simulink model "Forward_and_inverse_Both"  (R2024b)
settings: Solver=VariableStepAuto  StartTime=0.0  StopTime=7  MaxStep=0.005  RelTol=1e-3
model workspace: external: MATLAB File D:\OneDrive - itc.edu.kh\V4_robot_arm\Import_arm6\Test_Assembly_DataFile.m (data not in the file)
values from neighbouring files (symbols this model uses):
  Reach_max = max(REACH_MAX)    [Workspace_sample.m]
  Reach_min = max(REACH_MIN)    [Workspace_sample.m]
undefined symbols (not defined in the file or in its folder): DiscIntNeverNeededParam, initialPose, maxAngularAcc, maxAngularVel, maxLinearAcc, maxLinearVel, poseTol, smiData, Ts, wps1, X, Y, Z
libraries: sm_lib x140, nesl_utility x52, stmnucleolib x12, simulink x4, vrlib x2, vexcommonlib x2, robotcorelib x2
(part 6 of 6)

== matlab function Forward_and_inverse_Both/MATLAB Function ==
  data: Reach_min input; Reach_max input; x input; x_error input; x_out output; y input; y_error input; z input; z_error input; y_out output; z_out output; Out output
function [x_out, y_out, z_out, Out] = fcn(Reach_min, Reach_max, x, x_error, y, y_error, z, z_error)
    % Calculate the radial distance from origin
    Out = sqrt(x^2 + y^2 + z^2);

    % Check conditions for updating outputs
    if Out > Reach_min || Out < Reach_max || x == 0 && y == 0
        % Update outputs only if Out is within bounds and x, y = 0
        x_out = x;
        y_out = y;
        z_out = z;
    else
        % Retain previous outputs or use error positions
        x_out = x_error;
        y_out = y_error;
        z_out = z_error;
    end
end

== matlab function Forward_and_inverse_Both/Flip the state of a button1/MATLAB Function1 ==
  data: y output; X input; delta input; n input; error output
function [y , error] = fcn(X,delta,n)

    if X == 1 && n <= 2
        delta = 0;
        n = n + 1;
    elseif X == 1 && n > 2
        delta = 0;
        n = 0;
    elseif X == 0
        n = 0;
        delta = 1;
    end
    y = delta;
    error = n;
end

== matlab function Forward_and_inverse_Both/Set Delta for the joint movement more Delta, faster the movement1/ speed setting ==
  data: O input; Tri input; y output; delta input
function y = fcn(O,Tri,delta)

    if O == 1 && Tri ==0 && delta <= 0.1
        delta = delta + 0.025;
    elseif Tri == 1 && O == 0 && delta >= 0.025
        delta = delta - 0.025;
    else
    end
    y = delta;
end

== matlab function Forward_and_inverse_Both/Set Joint position to where it were left off1/Joint3 ==
  data: pos input; posfinal output; pos_prev input; delta input
function posfinal = fcn(pos,pos_prev,delta)

if pos > 0        %%In case of clockwise rotation
    posc = pos_prev + abs(delta);
elseif pos < 0    %%In case of counter clockwise rotation
    posc = pos_prev - abs(delta);
else               %%Stay still if there's no input
    posc = pos_prev;
end

if posc <= 1 && posc >= -1.2 %%The joint only update its position if it stays within this range
    posfinal = posc;
else
    posfinal = pos_prev;
end

== matlab function Forward_and_inverse_Both/Set Joint position to where it were left off1/Joint4 ==
  data: pos input; posfinal output; pos_prev input; delta input
function posfinal = fcn(pos,pos_prev,delta)

if pos > 0        %%In case of clockwise rotation
    posc = pos_prev + abs(delta);
elseif pos < 0    %%In case of counter clockwise rotation
    posc = pos_prev - abs(delta);
else               %%Stay still if there's no input
    posc = pos_prev;
end

if posc <= 1 && posc >= -1.2 %%The joint only update its position if it stays within this range
    posfinal = posc;
else
    posfinal = pos_prev;
end

== matlab function Forward_and_inverse_Both/Set Joint position to where it were left off1/MATLAB Function2 ==
  data: delta input; n input; y output; pos input; pos_prev input
function y = fcn(delta,n,pos,pos_prev)
if n == 0 && pos > 0
    pos = max(0,pos_prev - abs(delta));
elseif n == 0 && pos < 0
    pos = min(0,pos_prev + abs(delta));
end
y = pos;

== matlab function Forward_and_inverse_Both/Set Joint position to where it were left off1/MATLAB Function3 ==
  data: delta input; n input; y output; pos input; pos_prev input
function y = fcn(delta,n,pos,pos_prev)
if n == 0 && pos > 0
    pos = max(0,pos_prev - abs(delta));
elseif n == 0 && pos < 0
    pos = min(0,pos_prev + abs(delta));
end
y = pos;

== matlab function Forward_and_inverse_Both/Set Joint position to where it were left off1/limit J2 & J3 so that it won't collide with itself/Joint1 ==
  data: pos input; posfinal output; pos_prev input; delta input
function posfinal = fcn(pos,pos_prev,delta)

if pos > 0        %%In case of clockwise rotation
    posc = pos_prev + abs(delta);
elseif pos < 0    %%In case of counter clockwise rotation
    posc = pos_prev - abs(delta);
else               %%Stay still if there's no input
    posc = pos_prev;
end

if posc <= 1 && posc >= -1.2 %%The joint only update its position if it stays within this range
    posfinal = posc;
else
    posfinal = pos_prev;
end

== matlab function Forward_and_inverse_Both/Set Joint position to where it were left off1/limit J2 & J3 so that it won't collide with itself/Joint2 ==
  data: pos input; delta input; posfinal output; pos_prev input
function posfinal = fcn(pos,delta,pos_prev)

if pos > 0        %%In case of clockwise rotation
    posc = pos_prev + abs(delta);
elseif pos < 0    %%In case of counter clockwise rotation
    posc = pos_prev - abs(delta);
else               %%Stay still if there's no input
    posc = pos_prev;
end

if posc <= 1 && posc >= -1.2 %%The joint only update its position if it stays within this range
    posfinal = posc;
else
    posfinal = pos_prev;
end

== matlab function Forward_and_inverse_Both/Set Joint position to where it were left off1/limit J2 & J3 so that it won't collide with itself/MATLAB Function ==
  data: delta input; n input; y output; pos input; pos_prev input
function y = fcn(delta,n,pos,pos_prev)
if n == 0 && pos > 0
    pos = max(0,pos_prev - abs(delta));
elseif n == 0 && pos < 0
    pos = min(0,pos_prev + abs(delta));
end
y = pos;

== matlab function Forward_and_inverse_Both/Set Joint position to where it were left off1/limit J2 & J3 so that it won't collide with itself/MATLAB Function1 ==
  data: delta input; n input; y output; pos input; pos_prev input
function y = fcn(delta,n,pos,pos_prev)
if n == 0 && pos > 0
    pos = max(0,pos_prev - abs(delta));
elseif n == 0 && pos < 0
    pos = min(0,pos_prev + abs(delta));
end
y = pos;

== matlab function Forward_and_inverse_Both/Set Joint position to where it were left off1/limit J2 & J3 so that it won't collide with itself/MATLAB Function4 ==
  data: J2 input; J2_prev input; J3 input; J2final output; J3final output; J3_prev input
function [J2final, J3final] = fcn(J2, J2_prev, J3, J3_prev)
J2final = max(0.975,J3_prev + 0.725 < 0.05);
J3final = max(-0.725,J2_prev - 0.975 < 0.05);
end
J2final = J2;
J3final = J3;

== matlab function Forward_and_inverse_Both/Subsystem20/Joint 1 R1 = counter-clockwise L1 = clockwise/MATLAB Function1 ==
  data: buttonL input; buttonR input; pos output; pos_prev input; delta input
function pos = fcn(buttonL,buttonR, pos_prev,delta)

    if buttonR == 1 && buttonL == 0

        pos = pos_prev + delta;
    elseif buttonR == 0 && buttonL == 1
    
        pos = pos_prev - delta;
    else
        pos = pos_prev;
    end
end

== matlab function Forward_and_inverse_Both/Subsystem20/Joint 1 R1 = counter-clockwise L1 = clockwise/Position limiter ==
  data: pos input; delta input; y output
function y = fcn(pos,delta)

if pos <= -1.3
    pos = pos + delta; %pos = pos_prev
elseif pos >= 1.3
    pos = pos - delta;
end

y = pos;

== matlab function Forward_and_inverse_Both/Subsystem20/Joint 6 L = counter-clockwise R = clockwise/MATLAB Function1 ==
  data: buttonL input; buttonR input; pos output; pos_prev input; delta input
function pos = fcn(buttonL,buttonR, pos_prev,delta)

    if buttonR == 1 && buttonL == 0

        pos = pos_prev - delta*1.25;
    elseif buttonR == 0 && buttonL == 1
    
        pos = pos_prev + delta*1.25;
    else
        pos = pos_prev;
    end
end

== matlab function Forward_and_inverse_Both/Subsystem20/Joint 6 L = counter-clockwise R = clockwise/Position limiter ==
  data: pos input; delta input; y output
function y = fcn(pos,delta)

if pos <= -1.3
    pos = pos + delta; %pos = pos_prev
elseif pos >= 1.3
    pos = pos - delta;
end

y = pos;

== matlab function Forward_and_inverse_Both/Subsystem20/MATLAB Function ==
  data: delta input; n input; y output; pos input; pos_prev input
function y = fcn(delta,n,pos,pos_prev)
if n == 0 && pos > 0
    pos = max(0,pos_prev - abs(delta));
elseif n == 0 && pos < 0
    pos = min(0,pos_prev + abs(delta));
end
y = pos;

== matlab function Forward_and_inverse_Both/Subsystem20/MATLAB Function1 ==
  data: delta input; n input; y output; pos input; pos_prev input
function y = fcn(delta,n,pos,pos_prev)
if n == 0 && pos > 0
    pos = max(0,pos_prev - abs(delta));
elseif n == 0 && pos < 0
    pos = min(0,pos_prev + abs(delta));
end
y = pos;

== matlab function Forward_and_inverse_Both/Waypoint Trajectory/1st Order Filter ==
  data: Y_dot input; Y input; X input; Y_ddot output
function Y_ddot = fcn(Y_dot,Y,X)

Y_ddot = zeros(4,1);
zeta = 1;
wn = 2*pi*1;

Y_ddot(1) = (-wn*wn*Y(1) - 2*zeta*wn*Y_dot(1) + wn*wn*X(1));
Y_ddot(2) = (-wn*wn*Y(2) - 2*zeta*wn*Y_dot(2) + wn*wn*X(2));
Y_ddot(3) = (-wn*wn*Y(3) - 2*zeta*wn*Y_dot(3) + wn*wn*X(3));
Y_ddot(4) = (-wn*wn*Y(4) - 2*zeta*wn*Y_dot(4) + wn*wn*X(4));
